simulink model "StackForce_tricycle"  (R2019b)
settings: Solver=ode4  StartTime=0.0  StopTime=inf  FixedStep=0.002  RelTol=1e-3
libraries: xpcrtudplib x4, aerolibanimutils x1
settings Model: xpc_rtwmakecfg_data=_xpcnblib__xpcetherlib__xpcether8255xlib__xpcetherGbElib_  Creator=s336079  LastModifiedBy=M

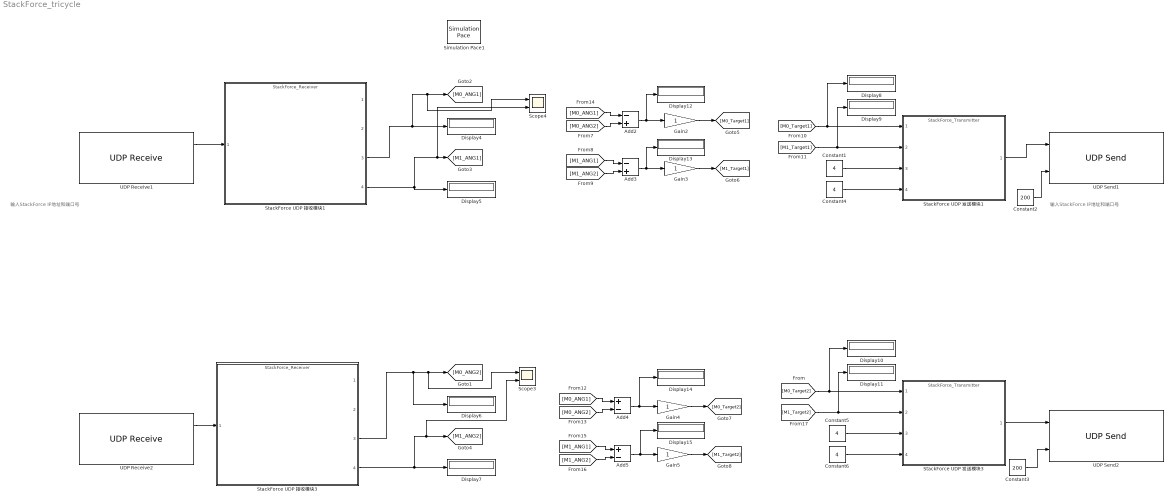
== system StackForce_tricycle ==
  note: 输入StackForce IP地址和端口号
  note: 输入StackForce IP地址和端口号
  Add2 : Sum  Inputs=-+
  Add3 : Sum  Inputs=-+
  Add4 : Sum  Inputs=+-
  Add5 : Sum  Inputs=+-
  Constant{1,4..6} (4 alike) : Constant  Value=4
  Constant2 : Constant  Value=200
  Constant3 : Constant  Value=200
  Display{4..15} (12 alike) : Display
  Gain{2..5} (4 alike) : Gain
  Scope3 : Scope  NumInputPorts=2
  Scope4 : Scope  NumInputPorts=2
  Simulation Pace1 : aerolibanimutils/Simulation Pace  SimulationPace=1  SleepMode=Auto  OutputPaceError=off  SampleTime=0.002
  StackForce UDP 发送模块1 : ModelReference  ModelNameDialog=StackForce_Transmitter  ModelReferenceVersion=1.493  CopyOfModelProtected=on
  StackForce UDP 发送模块3 : ModelReference  ModelNameDialog=StackForce_Transmitter  ModelReferenceVersion=1.493  CopyOfModelProtected=on
  StackForce UDP 接收模块1 : ModelReference  ModelNameDialog=StackForce_Receiver  ModelReferenceVersion=1.493  CopyOfModelProtected=on
  StackForce UDP 接收模块3 : ModelReference  ModelNameDialog=StackForce_Receiver  ModelReferenceVersion=1.493  CopyOfModelProtected=on
  UDP Receive1 : xpcrtudplib/UDP Receive  ipAddressVal=Use host-target connection  localPort=2310  rcvWidth=1024  rcvFmAny=off  fmAddress=192.168.10.212  rcvMulticast=off  multicastAddress={}  maxUDPQueue=8  sampleTime=-1
      settings: SourceProductName=Simulink Real-Time
  UDP Receive2 : xpcrtudplib/UDP Receive  ipAddressVal=Use host-target connection  localPort=2410  rcvWidth=1024  rcvFmAny=off  fmAddress=192.168.10.214  rcvMulticast=off  multicastAddress={}  maxUDPQueue=8  sampleTime=-1
      settings: SourceProductName=Simulink Real-Time
  UDP Send1 : xpcrtudplib/UDP Send  ipAddressVal=Use host-target connection  localPort=25001  toAddress=192.168.10.212  toPort=2310  sampleTime=-1
      settings: SourceProductName=Simulink Real-Time  SourceProductBaseCode=XP
  UDP Send2 : xpcrtudplib/UDP Send  ipAddressVal=Use host-target connection  localPort=25002  toAddress=192.168.10.214  toPort=2410  sampleTime=-1
      settings: SourceProductName=Simulink Real-Time  SourceProductBaseCode=XP
  wires:
  Add2/1 -> Display12/1, Gain2/1
  Add3/1 -> Display13/1, Gain3/1
  [M0_ANG1] -> Add2/1
  [M0_ANG2] -> Add2/2
  Gain2/1 -> [M0_Target1]
  [M1_ANG2] -> Add3/2
  [M1_ANG1] -> Add3/1
  [M0_Target1] -> StackForce UDP 发送模块1/1, Display8/1
  Gain3/1 -> [M1_Target1]
  [M1_Target1] -> StackForce UDP 发送模块1/2, Display9/1
  [M0_ANG2] -> Add4/2
  Add5/1 -> Display15/1, Gain5/1
  Gain5/1 -> [M1_Target2]
  [M1_ANG2] -> Add5/2
  [M1_ANG1] -> Add5/1
  [M0_ANG1] -> Add4/1
  Add4/1 -> Display14/1, Gain4/1
  Gain4/1 -> [M0_Target2]
  [M0_Target2] -> StackForce UDP 发送模块3/1, Display10/1
  [M1_Target2] -> StackForce UDP 发送模块3/2, Display11/1
  Constant1/1 -> StackForce UDP 发送模块1/3
  Constant4/1 -> StackForce UDP 发送模块1/4
  Constant6/1 -> StackForce UDP 发送模块3/4
  Constant5/1 -> StackForce UDP 发送模块3/3
  StackForce UDP 接收模块1/3 -> Scope4/1, [M0_ANG1], Display4/1
  StackForce UDP 接收模块1/4 -> Display5/1, Scope4/2, [M1_ANG1]
  StackForce UDP 接收模块3/4 -> Scope3/2, [M1_ANG2], Display7/1
  StackForce UDP 接收模块3/3 -> Display6/1, Scope3/1, [M0_ANG2]
  UDP Receive2/1 -> StackForce UDP 接收模块3/1
  UDP Receive1/1 -> StackForce UDP 接收模块1/1
  StackForce UDP 发送模块1/1 -> UDP Send1/1
  StackForce UDP 发送模块3/1 -> UDP Send2/1
  Constant2/1 -> UDP Send1/2
  Constant3/1 -> UDP Send2/2
